simulink model "demo3"  (R2020a)
settings: Solver=FixedStepAuto  StartTime=0.0  StopTime=2  FixedStep=0.2  RelTol=1e-3
settings Model: Creator=nikhil  LastModifiedBy=nikhil

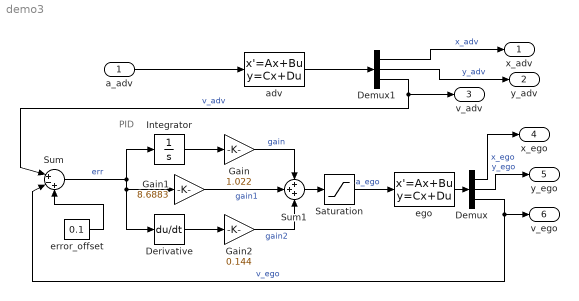
== system demo3 ==
  note: PID
  a_adv : Inport
  Demux : Demux  Outputs=3
  Demux1 : Demux  Outputs=3
  Derivative : Derivative
  Gain : Gain  Gain=1.022
  Gain1 : Gain  Gain=8.6883
  Gain2 : Gain  Gain=0.144
  Integrator : Integrator  InitialCondition=0.001
  Saturation : Saturate  UpperLimit=15  LowerLimit=-15  ZeroCross=off
  Sum : Sum  Inputs=|+-+
  Sum1 : Sum  Inputs=+++
  adv : StateSpace  A=[0 0 1 ; 0 0 0; 0 0 0]  B=[0; 0; 1]  C=[1 0 0;0 1 0; 0 0 1]  D=zeros(3,1)  InitialCondition=[-1;0;0]
  ego : StateSpace  A=[0 0 0 ; 0 0 1; 0 0 0]  B=[0; 0; 1]  C=[1 0 0 ; 0 1 0; 0 0 1]  D=zeros(3,1)  InitialCondition=[0; -1; 0];
  error_offset : Constant  Value=0.1
  x_adv : Outport
  y_adv : Outport  Port=2
  v_adv : Outport  Port=3
  x_ego : Outport  Port=4
  y_ego : Outport  Port=5
  v_ego : Outport  Port=6
  wires:
  ego/1 -> Demux/1
  a_adv/1 -> adv/1
  adv/1 -> Demux1/1
  Demux/1 -> x_ego/1  "x_ego"
  Demux/2 -> y_ego/1  "y_ego"
  Demux/3 -> Sum/2, v_ego/1  "v_ego"
  Demux1/1 -> x_adv/1  "x_adv"
  Demux1/2 -> y_adv/1  "y_adv"
  Demux1/3 -> Sum/1, v_adv/1  "v_adv"
  Sum/1 -> Derivative/1, Gain1/1, Integrator/1  "err"
  Gain/1 -> Sum1/1  "gain"
  Gain2/1 -> Sum1/3  "gain2"
  Integrator/1 -> Gain/1
  Sum1/1 -> Saturation/1
  Derivative/1 -> Gain2/1
  Saturation/1 -> ego/1  "a_ego"
  Gain1/1 -> Sum1/2  "gain1"
  error_offset/1 -> Sum/3
